simulink model "LAB4_TELEMETRY_2023b"  (R2023b)
settings: Solver=FixedStepAuto  StartTime=0.0  StopTime=1  RelTol=1e-8
undefined symbols (not defined in the file): CR, LF
libraries: instrumentseriallib x2
settings Model: Creator=anton  LastModifiedBy=admin
settings DataIOCC: ExternalInput=data
settings OptimizationCC: ReuseModelBlockBuffer=off
settings DebuggingCC: ParameterPrecisionLossMsg=none

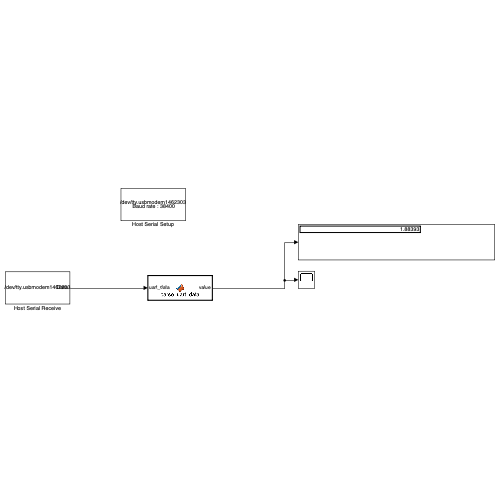
[thumbnail: Simulink's stored preview of the top-level diagram]
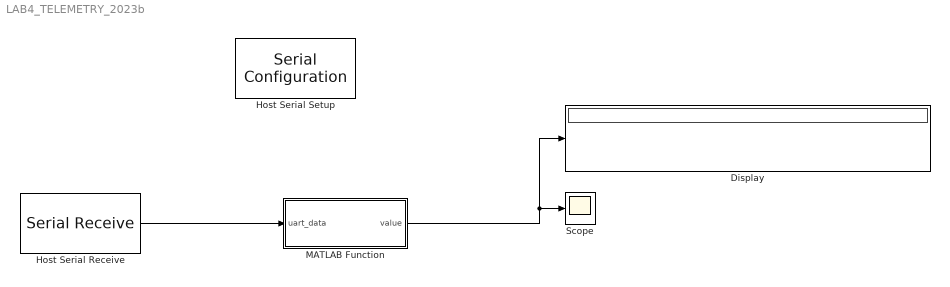
== system LAB4_TELEMETRY_2023b ==
  Display : Display
  Host Serial Receive : instrumentseriallib/Serial Receive  PortSel=/dev/tty.usbmodem1462303  Port=/dev/tty.usbmodem1462303  ComPort=/dev/tty.usbmodem1462303  DataType=uint8  SaveDataType=uint8  ToggleHeader=on  Header=['v=']  ToggleTerminator=off  Terminator=CR/LF ('\r\n')  CustomTerminator='E'  InputFormat=Column major  ToggleDataSize=on  DataSize=[8 1]  EnableBlockingMode=on  ActionDataUnavailable=Error  ActionWhenDataUnavailable=Error  CustomValue=5  SampleTime=0.001  SimulateUsing=Interpreted execution  BlockInModel=on  aMode=5
      settings: LibrarySourceBlock=mcblib/Protection and Diagnostics/Host Serial Receive
  Host Serial Setup : instrumentseriallib/Serial Configuration  Priority=-99  PortSel=/dev/tty.usbmodem1462303  Port=/dev/tty.usbmodem1462303  ComPort=/dev/tty.usbmodem1462303  BaudRate=38400  DataBits=8  Parity=none  StopBits=1  ByteOrder=little-endian  FlowControl=none  Timeout=10  SimulateUsing=Interpreted execution  BlockInModel=on  aMode=5
      settings: LibrarySourceBlock=mcblib/Protection and Diagnostics/Host Serial Setup
  MATLAB Function : MATLAB Function  TreatAsAtomicUnit=on
  Scope : Scope
  wires:
  Host Serial Receive/1 -> MATLAB Function/1(uart_data)
  MATLAB Function/1(value) -> Display/1, Scope/1

== matlab function LAB4_TELEMETRY_2023b/MATLAB Function ==
  data: uart_data input; value output
function value = parse_uart_data(uart_data)
    str = char(uart_data');
    value = str2double(str);
    disp(str);
    disp('-----');
end
